simulink model "35 Bus Network Electricity Transmission Model"  (R2023b)
settings: Solver=VariableStepAuto  StartTime=0.0  StopTime=1  RelTol=1e-3
model workspace (MAT data in the model file):
  T_set = 0.0001
  Tp = 5e-05
undefined symbols (not defined in the file): D1, D11, Delta, DiscIntNeverNeededParam
libraries: spsSeriesRLCBranchLib x57, spsLoadFlowBusLib x35, spsThreePhaseSeriesRLCLoadLib x28, spsThreePhaseTransformerTwoWindingsLib x22, spsDistributedParametersLineLib x22, spsGenericPowerSystemStabilizerLib x20, spsThreePhaseVIMeasurementLib x14, spsSynchronousMachinepuStandardLib x10, spsExcitationSystemLib x10, spsHydraulicTurbineandGovernorLib x10, spsFourierLib x8, spsMeanLib x8
(part 3 of 8)

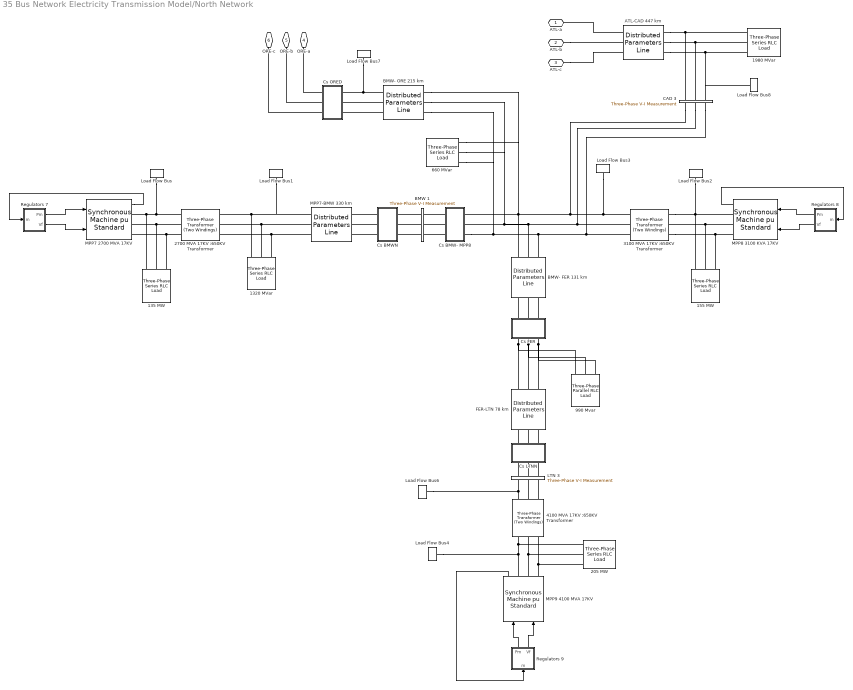
== system 35 Bus Network Electricity Transmission Model/North Network ==
  1320 MVar : spsThreePhaseSeriesRLCLoadLib/Three-Phase Series RLC Load  LConnTagsString=A|B|C  Configuration=Y (grounded)  NominalVoltage=650e3  Vabc=[1e3 1e3 1e3]  Vabcp=[1e3 1e3 1e3]  NominalFrequency=60  UnbalancedPower=off  ActivePower=4400e3  InductivePower=1320e6  CapacitivePower=0  Pabc=[10e3 9e3 11e3]  QLabc=[100 90 110]  QCabc=[100 90 110]  Pabcp=[10e3 9e3 11e3]  QLabcp=[100 90 110]  QCabcp=[100 90 110]  Measurements=None  LoadType=constant Z
  135 MW : spsThreePhaseSeriesRLCLoadLib/Three-Phase Series RLC Load  LConnTagsString=A|B|C  Configuration=Y (grounded)  NominalVoltage=17e3  Vabc=[1e3 1e3 1e3]  Vabcp=[1e3 1e3 1e3]  NominalFrequency=60  UnbalancedPower=off  ActivePower=135e6  InductivePower=0  CapacitivePower=0  Pabc=[10e3 9e3 11e3]  QLabc=[100 90 110]  QCabc=[100 90 110]  Pabcp=[10e3 9e3 11e3]  QLabcp=[100 90 110]  QCabcp=[100 90 110]  Measurements=None  LoadType=constant Z
  155 MW : spsThreePhaseSeriesRLCLoadLib/Three-Phase Series RLC Load  LConnTagsString=A|B|C  Configuration=Y (grounded)  NominalVoltage=17e3  Vabc=[1e3 1e3 1e3]  Vabcp=[1e3 1e3 1e3]  NominalFrequency=60  UnbalancedPower=off  ActivePower=155e6  InductivePower=0  CapacitivePower=0  Pabc=[10e3 9e3 11e3]  QLabc=[100 90 110]  QCabc=[100 90 110]  Pabcp=[10e3 9e3 11e3]  QLabcp=[100 90 110]  QCabcp=[100 90 110]  Measurements=None  LoadType=constant Z
  1980 MVar : spsThreePhaseSeriesRLCLoadLib/Three-Phase Series RLC Load  LConnTagsString=A|B|C  Configuration=Y (grounded)  NominalVoltage=650e3  Vabc=[1e3 1e3 1e3]  Vabcp=[1e3 1e3 1e3]  NominalFrequency=60  UnbalancedPower=off  ActivePower=6600e3  InductivePower=1980e6  CapacitivePower=0  Pabc=[10e3 9e3 11e3]  QLabc=[100 90 110]  QCabc=[100 90 110]  Pabcp=[10e3 9e3 11e3]  QLabcp=[100 90 110]  QCabcp=[100 90 110]  Measurements=None  LoadType=constant Z
  205 MW : spsThreePhaseSeriesRLCLoadLib/Three-Phase Series RLC Load  LConnTagsString=A|B|C  Configuration=Y (grounded)  NominalVoltage=17e3  Vabc=[1e3 1e3 1e3]  Vabcp=[1e3 1e3 1e3]  NominalFrequency=60  UnbalancedPower=off  ActivePower=205e6  InductivePower=0  CapacitivePower=0  Pabc=[10e3 9e3 11e3]  QLabc=[100 90 110]  QCabc=[100 90 110]  Pabcp=[10e3 9e3 11e3]  QLabcp=[100 90 110]  QCabcp=[100 90 110]  Measurements=None  LoadType=constant Z
  "2700 MVA 17KV :650KV Transformer " : spsThreePhaseTransformerTwoWindingsLib/Three-Phase Transformer (Two Windings)  Winding1Connection=Yg  Winding2Connection=Delta (D1)  CoreType=Three single-phase transformers  SetSaturation=off  Hysteresis=off  DataFile='hysteresis'  SetInitialFlux=off  Measurements=None  UNITS=pu  NominalPower=[ 2700e6 , 60 ]  Winding1=[650e3 , 0.002 , 0.08 ]  Winding2=[17e3 , 0.002 , 0.08 ]  Rm=500  Lm=500  L0=0.5  Saturation=[ 0,0 ; 0.0024,1.2 ; 1.0,1.52 ]  InitialFluxes=[ 0.8 , -0.8 , 0.7 ]  BreakLoop=off  DiscreteSolver=Trapezoidal iterative  DataType=off  TransfoNumber=1
  "3100 MVA 17KV :650KV Transformer " : spsThreePhaseTransformerTwoWindingsLib/Three-Phase Transformer (Two Windings)  Winding1Connection=Yg  Winding2Connection=Delta (D1)  CoreType=Three single-phase transformers  SetSaturation=off  Hysteresis=off  DataFile='hysteresis'  SetInitialFlux=off  Measurements=None  UNITS=pu  NominalPower=[ 3100e6 , 60 ]  Winding1=[ 650e3 , 0.002 , 0.08 ]  Winding2=[ 17e3 , 0.002 , 0.08 ]  Rm=500  Lm=500  L0=0.5  Saturation=[ 0,0 ; 0.0024,1.2 ; 1.0,1.52 ]  InitialFluxes=[ 0.8 , -0.8 , 0.7 ]  BreakLoop=off  DiscreteSolver=Trapezoidal iterative  DataType=off  TransfoNumber=1
  "4100 MVA 17KV :650KV Transformer " : spsThreePhaseTransformerTwoWindingsLib/Three-Phase Transformer (Two Windings)  Winding1Connection=Yg  Winding2Connection=Delta (D1)  CoreType=Three single-phase transformers  SetSaturation=off  Hysteresis=off  DataFile='hysteresis'  SetInitialFlux=off  Measurements=None  UNITS=pu  NominalPower=[ 4100e6 , 60 ]  Winding1=[ 650e3 , 0.002 , 0.08 ]  Winding2=[ 17e3 , 0.002 , 0.08 ]  Rm=500  Lm=500  L0=0.5  Saturation=[ 0,0 ; 0.0024,1.2 ; 1.0,1.52 ]  InitialFluxes=[ 0.8 , -0.8 , 0.7 ]  BreakLoop=off  DiscreteSolver=Trapezoidal iterative  DataType=off  TransfoNumber=1
  660 MVar : spsThreePhaseSeriesRLCLoadLib/Three-Phase Series RLC Load  LConnTagsString=A|B|C  Configuration=Y (grounded)  NominalVoltage=650e3  Vabc=[1e3 1e3 1e3]  Vabcp=[1e3 1e3 1e3]  NominalFrequency=60  UnbalancedPower=off  ActivePower=2200e3  InductivePower=660e6  CapacitivePower=0  Pabc=[10e3 9e3 11e3]  QLabc=[100 90 110]  QCabc=[100 90 110]  Pabcp=[10e3 9e3 11e3]  QLabcp=[100 90 110]  QCabcp=[100 90 110]  Measurements=None  LoadType=constant Z
  990 Mvar : spsThreePhaseParallelRLCLoadLib/Three-Phase Parallel RLC Load  LConnTagsString=A|B|C  Configuration=Y (grounded)  NominalVoltage=650e3  Vabc=[1e3 1e3 1e3]  Vabcp=[1e3 1e3 1e3]  NominalFrequency=60  UnbalancedPower=off  ActivePower=3300e3  InductivePower=990e6  CapacitivePower=0  Pabc=[10e3 9e3 11e3]  QLabc=[100 90 110]  QCabc=[100 90 110]  Pabcp=[10e3 9e3 11e3]  QLabcp=[100 90 110]  QCabcp=[100 90 110]  Measurements=None  LoadType=constant Z
  ATL-CAD 447 km : spsDistributedParametersLineLib/Distributed Parameters Line  Phases=3  Length=447  Frequency=60  Resistance=[0.01273 0.3864]/6  Inductance="[0.9337e-3  4.1264e-3]/6"  Capacitance=[12.74e-9 7.751e-9]*6  x1=[-0.00258 -5.31602971925857e-09 -148199.916502334 -96849.1917886608;-0.00252 -6.01655285993135e-09 -145971.498172148 -100176.353662668;-0.00246 -6.71399782098787e-09 -143668.398126254 -103452.263463096;-0.0024 -7.40800777669876e-09 -141291.794673192 -106675.245173957;-0.00234 -8.09822765874685e-09 -138842.903727203 -109843.649858256;-0.00228 -8.78430433788667e-09 -136322.978186145 -112955.85650161;-0.00222 -9.46588680461196e-09 -133733.307290488 -116010.272841594;-0.00216 -1.01426263487385e-08 -131075.215963714 -119005.336182368;-0.0021 -1.08141767378109e-08 -128350.064134461 -121939.514194186;-0.00204 -1.14801943942412e-08 -125559.246040761 -124811.305697358;-0.00198 -1.21403385710898e-08 -122704.189516718 -127619.241430289;-0.00192 -1.27942715263977e-08 -119786.355262006 -130361.884801171;-0.00186 -1.34416586959818e-08 -116807.236094544 -133037.832622978;-0.0018 -1.40821688646038e-08 -113768.356186747 -135645.715831359;-0.00174 -1.4715474335426e-08 -110671.270285727 -138184.200185075;-0.00168 -1.53412510976676e-08 -107517.562917858 -140651.986948627;-0.00162 -1.59591789923738e-08 -104308.847578105 -143047.813556706;-0.00156 -1.65689418762158e-08 -101046.765904525 -145370.454260149;-0.0015 -1.71702277832351e-08 -97732.9868383792 -147618.720753056;-0.00144 -1.77627290844512e-08 -94369.2057702685 -149791.462780745;-0.00138 -1.83461426452502e-08 -90957.1436727434 -151887.568728248;-0.00132 -1.89201699804741e-08 -87498.5462198204 -153905.96618903;-0.00126 -1.94845174071315e-08 -83995.1828938642 -155845.622513654;-0.0012 -2.00388961946509e-08 -80448.8460802869 -157705.545338104;-0.00114 -2.05830227126009e-08 -76861.3501505312 -159484.783091496;-0.00108 -2.11166185758005e-08 -73234.530533804 -161182.425482918;-0.00102 -2.16394107867466e-08 -69570.2427780372 -162797.603967154;-0.00096 -2.21511318752838e-08 -65870.3616005549 -164329.492189047;-0.0009 -2.26515200354478e-08 -62136.7799289334 -165777.306406276;-0.00084 -2.31403192594097e-08 -58371.4079325445 -167140.305890335;-0.00078 -2.36172794684545e-08 -54576.1720452778 -168417.793305503;-0.00072 -2.40821566409261e-08 -50753.013979941 -169609.115065613;-0.00066 -2.45347129370731e-08 -46903.8897348442 -170713.661668439;-0.0006 -2.49747168207321e-08 -43030.7685930748 -171730.86800753;-0.00054 -2.5401943177786e-08 -39135.632114976 -172660.213661326;-0.00048 -2.58161734313361e-08 -35220.4731243439 -173501.22315942;-0.00042 -2.62171956535308e-08 -31287.2946888618 -174253.466225811;-0.00036 -2.6604804673991e-08 -27338.1090952941 -174916.557999047;-0.0003 -2.69788021847797e-08 -23374.9368199632 -175490.159229125;-0.00024 -2.73389968418598e-08 -19399.8054950359 -175973.976451055;-0.00018 -2.7685204362989e-08 -15414.7488711503 -176367.762135008;-0.00012 -2.80172476220023e-08 -11421.8057769103 -176671.314812951;-6e-05 -2.8334956739433e-08 -7423.01907578413 -176884.479181725]  x2=[-0.00258 -4.87845949451141e-08 -272951.515548649 -95064.3825346825;-0.00252 -4.87524641140646e-08 -270731.542277713 -101213.579527017;-0.00246 -4.86953906215323e-08 -268373.057747203 -107310.993781853;-0.0024 -4.86134036673707e-08 -265877.268601386 -113353.505749391;-0.00234 -4.85065451976205e-08 -263245.451732106 -119338.023968856;-0.00228 -4.83748698830492e-08 -260478.953625503 -125261.486650145;-0.00222 -4.8218445091181e-08 -257579.189673127 -131120.863240298;-0.00216 -4.80373508518297e-08 -254547.643447798 -136913.155973982;-0.0021 -4.78316798161544e-08 -251385.865944582 -142635.401407206;-0.00204 -4.76015372092573e-08 -248095.474787272 -148284.67193347;-0.00198 -4.73470407763487e-08 -244678.153400783 -153858.077281588;-0.00192 -4.70683207225062e-08 -241135.650149882 -159352.765994398;-0.00186 -4.67655196460595e-08 -237469.77744469 -164765.926887624;-0.0018 -4.64387924656344e-08 -233682.41081342 -170094.790488131;-0.00174 -4.60883063408937e-08 -229775.487942824 -175336.630450834;-0.00168 -4.5714240587015e-08 -225751.007686833 -180488.764953549;-0.00162 -4.53167865829499e-08 -221611.02904391 -185548.558069065;-0.00156 -4.48961476735111e-08 -217357.670103628 -190513.421113731;-0.0015 -4.44525390653371e-08 -212993.106963013 -195380.813971871;-0.00144 -4.39861877167887e-08 -208519.572613215 -200148.24639536;-0.00138 -4.34973322218332e-08 -203939.35579707 -204813.27927768;-0.00132 -4.29862226879746e-08 -199254.799838133 -209373.525901806;-0.00126 -4.24531206082949e-08 -194468.301441793 -213826.653161304;-0.0012 -4.18982987276684e-08 -189582.309469075 -218170.382753982;-0.00114 -4.13220409032214e-08 -184599.323683754 -222402.492347517;-0.00108 -4.07246419591047e-08 -179521.893473433 -226520.816716443;-0.00102 -4.01064075356569e-08 -174352.616545228 -230523.248849912;-0.00096 -3.94676539330326e-08 -169094.137596732 -234407.74102969;-0.0009 -3.88087079493778e-08 -163749.146962942 -238172.305877801;-0.00084 -3.81299067136336e-08 -158320.379239828 -241815.017373306;-0.00078 -3.74315975130551e-08 -152810.611885272 -245334.011837695;-0.00072 -3.67141376155325e-08 -147222.66379806 -248727.488888376;-0.00066 -3.59778940868065e-08 -141559.393875686 -251993.712359787;-0.0006 -3.52232436026707e-08 -135823.699551689 -255131.011191646;-0.00054 -3.4450572256257e-08 -130018.515313268 -258137.7802839;-0.00048 -3.36602753605036e-08 -124146.811199946 -261012.481317923;-0.00042 -3.28527572459055e-08 -118211.591284045 -263753.643543548;-0.00036 -3.20284310536511e-08 -112215.892133745 -266359.864531529;-0.0003 -3.11877185242524e-08 -106162.781259517 -268829.810891052;-0.00024 -3.03310497817739e-08 -100055.355544735 -271162.218951918;-0.00018 -2.94588631137736e-08 -93896.739661245 -273355.895411067;-0.00012 -2.85716047470672e-08 -87690.0844707324 -275409.717943088;-6e-05 -2.76697286194296e-08 -81438.5654126781 -277322.635774423]  x3=[-0.00258 -2.63643710027556e-10 -3962.84356104863 3839.79887558329;-0.00252 -2.75977166927134e-10 -4048.67593368483 3749.18694624542;-0.00246 -2.8816942880864e-10 -4132.43692890242 3656.65686358885;-0.0024 -3.00214257885608e-10 -4214.08369302854 3562.25596771361;-0.00234 -3.12105491800921e-10 -4293.57445406998 3466.03255586237;-0.00228 -3.23837046779582e-10 -4370.86854308459 3368.03585771063;-0.00222 -3.3540292074129e-10 -4445.92641498819 3268.31601017994;-0.00216 -3.46797196371213e-10 -4518.70966878661 3166.92403178691;-0.0021 -3.58014044147398e-10 -4589.18106722233 3063.91179654118;-0.00204 -3.69047725323257e-10 -4657.30455582573 2959.33200740577;-0.00198 -3.79892594863624e-10 -4723.04528136129 2853.23816933319;-0.00192 -3.9054310433285e-10 -4786.36960965905 2745.68456189141;-0.00186 -4.00993804733492e-10 -4847.24514282257 2636.72621149335;-0.0018 -4.11239349294119e-10 -4905.64073580424 2526.41886324438;-0.00174 -4.21274496204818e-10 -4961.52651233964 2414.81895242213;-0.00168 -4.31094111299001e-10 -5014.87388023287 2301.9835756031;-0.00162 -4.4069317068014e-10 -5065.65554598475 2187.97046145102;-0.00156 -4.50066763292085e-10 -5113.84552875675 2072.83794118182;-0.0015 -4.59210093431653e-10 -5159.41917366325 1956.64491872026;-0.00144 -4.68118483202194e-10 -5202.35316438539 1839.45084056365;-0.00138 -4.76787374906894e-10 -5242.62553510019 1721.31566536786;-0.00132 -4.85212333380574e-10 -5280.21568171866 1602.29983327142;-0.00126 -4.93389048258803e-10 -5315.10437242719 1482.46423497317;-0.0012 -5.01313336183161e-10 -5347.27375752696 1361.87018057953;-0.00114 -5.08981142941523e-10 -5376.70737856611 1240.57936823703;-0.00108 -5.16388545542266e-10 -5403.39017676026 1118.65385256647;-0.00102 -5.23531754221346e-10 -5427.30850069681 996.156012914591;-0.00096 -5.30407114381212e-10 -5448.45011331927 873.148521439658;-0.0009 -5.37011108460564e-10 -5466.80419818797 749.694311047227;-0.00084 -5.43340357734003e-10 -5482.36136501396 625.856543192506;-0.00078 -5.4939162404065e-10 -5495.11365446321 501.698575565788;-0.00072 -5.55161811440848e-10 -5505.05454222881 377.283929677488;-0.00066 -5.60647967800102e-10 -5512.1789423689 252.676258359358;-0.0006 -5.65847286299446e-10 -5516.48320990871 127.939313198532;-0.00054 -5.70757106871463e-10 -5517.96514270545 3.13691192102679;-0.00048 -5.75374917561226e-10 -5516.6239825749 -121.667094258581;-0.00042 -5.79698355811459e-10 -5512.46041567938 -246.408853304616;-0.00036 -5.83725209671265e-10 -5505.47657217664 -371.024545028189;-0.0003 -5.87453418927801e-10 -5495.67602513006 -495.45041373878;-0.00024 -5.90881076160322e-10 -5483.06378868061 -619.622800862831;-0.00018 -5.94006427716053e-10 -5467.6463154815 -743.478177512648;-0.00012 -5.96827874607388e-10 -5449.43149339691 -866.953176988952;-6e-05 -5.99343973329962e-10 -5428.42864146637 -989.984627200456]  x4=[-0.00258 1.25550589079962e-11 -6479.77720814425 -5262.43401290687;-0.00252 1.56860264672874e-11 -6359.09575517457 -5407.6451916609;-0.00246 1.88089687655935e-11 -6235.16087131396 -5550.08971921309;-0.0024 2.19222880479294e-11 -6108.03596393906 -5689.69471831107;-0.00234 2.50243914826226e-11 -5977.78607250148 -5826.38876445768;-0.00228 2.81136919762357e-11 -5844.47783525243 -5960.10192245311;-0.00222 3.11886089855525e-11 -5708.17945514932 -6090.765782175;-0.00216 3.42475693262131e-11 -5568.96066496193 -6218.31349357831;-0.0021 3.7289007977584e-11 -5426.89269159579 -6342.67980089709;-0.00204 4.0311368883452e-11 -5282.04821965117 -6463.80107603048;-0.00198 4.33131057481307e-11 -5134.50135423636 -6581.61535109605;-0.00192 4.62926828275745e-11 -4984.32758305404 -6696.06235013374;-0.00186 4.92485757150933e-11 -4831.60373778045 -6807.0835199441;-0.0018 5.21792721212672e-11 -4676.40795475683 -6914.62206004521;-0.00174 5.50832726476618e-11 -4518.81963501348 -7018.62295173288;-0.00168 5.7959091553948e-11 -4358.91940364667 -7119.0329862292;-0.00162 6.08052575180343e-11 -4196.78906856938 -7215.80079190516;-0.00156 6.36203143888224e-11 -4032.51157865687 -7308.87686056331;-0.0015 6.64028219312009e-11 -3866.17098130847 -7398.21357276708;-0.00144 6.91513565628964e-11 -3697.85237944741 -7483.76522220376;-0.00138 7.18645120828041e-11 -3527.64188798056 -7565.48803906867;-0.00132 7.45409003904268e-11 -3355.6265897405 -7643.34021245865;-0.00126 7.71791521960522e-11 -3181.89449093227 -7717.28191176325;-0.0012 7.97779177213074e-11 -3006.53447610784 -7787.27530704281;-0.00114 8.23358673897299e-11 -2829.63626269106 -7853.28458838299;-0.00108 8.4851692507004e-11 -2651.29035507662 -7915.27598421574;-0.00102 8.73241059305124e-11 -2471.58799832631 -7973.21777859748;-0.00096 8.97518427278629e-11 -2290.62113148636 -8027.08032743556;-0.0009 9.21336608240504e-11 -2108.48234054972 -8076.83607365474;-0.00084 9.4468341636926e-11 -1925.26481108739 -8122.45956129586;-0.00078 9.67546907006459e-11 -1741.06228057291 -8163.92744853963;-0.00072 9.89915382767822e-11 -1555.96899042455 -8201.21851964869;-0.00066 1.01177739952783e-10 -1370.07963778969 -8234.31369582201;-0.0006 1.03312177227474e-10 -1183.48932709597 -8263.19604495592;-0.00054 1.05393758083306e-10 -996.293521394147 -8287.85079030692;-0.00048 1.0742141754505e-10 -808.587993517389 -8308.26531805173;-0.00042 1.09394118224658e-10 -620.468777082158 -8324.42918374073;-0.00036 1.11310850852011e-10 -432.032117355627 -8336.33411764156;-0.0003 1.13170634791281e-10 -243.374422014822 -8343.97402897006;-0.00024 1.14972518542639e-10 -54.5922118226712 -8347.34500900643;-0.00018 1.16715580229062e-10 134.217928753796 -8346.44533309499;-0.00012 1.18398928067984e-10 322.95940095785 -8341.27546152656;-6e-05 1.20021700827546e-10 511.535641164771 -8331.83803930296]  x5=0.00252797080447097  V1=[6.404e-19 2.341e-08 2.341e-08;377 377 377;-1.588 0.8733 -0.6975]  V2=[3.447e-16 8.016e-05 8.016e-05;377 377 377;2.581 0.8892 -0.6816]  I1=[4.995e-19 5.332e-07 5.332e-07;377 377 377;1.203 -0.6479 -2.219]  I2=[4.022e-19 5.225e-07 5.225e-07;377 377 377;-2.95 1.909 0.3385]  nHarmo=1  Measurements=None  Decoupling=off  VsMag0=0  VrMag0=0  VsAngle0=0  VrAngle0=0  IsMag0=0  IrMag0=0  IsAngle0=0  IrAngle0=0
      settings: LibrarySourceBlock=sps_lib/Power Grid Elements/Distributed Parameters Line
  BMW 1 : spsThreePhaseVIMeasurementLib/Three-Phase V-I Measurement  VoltageMeasurement=no  SetLabelV=off  LabelV=Vabc  Vpu=off  VpuLL=off  CurrentMeasurement=no  SetLabelI=off  LabelI=Iabc  Ipu=off  Pbase=100e6  Vbase=500e3  OutputType=Complex  PhasorSimulation=off  PSBequivalent=0
  BMW- FER 131 km : spsDistributedParametersLineLib/Distributed Parameters Line  Phases=3  Length=131  Frequency=60  Resistance=[0.01273 0.3864]/6  Inductance="[0.9337e-3  4.1264e-3]/6"  Capacitance=[12.74e-9 7.751e-9]*6  x1=[-0.00078 -2.36172794684545e-08 -54576.1720452778 -168417.793305503;-0.00072 -2.40821566409261e-08 -50753.013979941 -169609.115065613;-0.00066 -2.45347129370731e-08 -46903.8897348442 -170713.661668439;-0.0006 -2.49747168207321e-08 -43030.7685930748 -171730.86800753;-0.00054 -2.5401943177786e-08 -39135.632114976 -172660.213661326;-0.00048 -2.58161734313361e-08 -35220.4731243439 -173501.22315942;-0.00042 -2.62171956535308e-08 -31287.2946888618 -174253.466225811;-0.00036 -2.6604804673991e-08 -27338.1090952941 -174916.557999047;-0.0003 -2.69788021847797e-08 -23374.9368199632 -175490.159229125;-0.00024 -2.73389968418598e-08 -19399.8054950359 -175973.976451055;-0.00018 -2.7685204362989e-08 -15414.7488711503 -176367.762135008;-0.00012 -2.80172476220023e-08 -11421.8057769103 -176671.314812951;-6e-05 -2.8334956739433e-08 -7423.01907578413 -176884.479181725]  x2=[-0.00078 -3.00128995055536e-08 -18133.3222512837 -146952.987792149;-0.00072 -3.02085545374644e-08 -14804.9695526073 -147325.549479172;-0.00066 -3.03887543146839e-08 -11469.0423579434 -147622.736692817;-0.0006 -3.05534066436764e-08 -8127.24738928558 -147844.397386617;-0.00054 -3.0702427285268e-08 -4781.29437068918 -147990.418154863;-0.00048 -3.08357399977448e-08 -1432.89515354457 -148060.724290632;-0.00042 -3.09532765758598e-08 1916.23715923744 -148055.279824007;-0.00036 -3.10549768857278e-08 5264.38908968081 -147974.087540477;-0.0003 -3.1140788895591e-08 8609.84766139116 -147817.188979514;-0.00024 -3.12106687024397e-08 11950.9012759463 -147584.664413322;-0.00018 -3.12645805544733e-08 15285.8405885813 -147276.632805765;-0.00012 -3.13024968693923e-08 18612.9593827214 -146893.251751505;-6e-05 -3.13243982485092e-08 21930.5554429133 -146434.717395374]  x3=[-0.00078 -5.25941512392795e-10 1443.1371085866 -8256.16688772562;-0.00072 -5.32217136019589e-10 1629.50173084287 -8221.41547476303;-0.00066 -5.38220467525353e-10 1815.03266990392 -8182.45783372926;-0.0006 -5.43948435494761e-10 1999.6350047131 -8139.31389607332;-0.00054 -5.49398109393558e-10 2183.21428930486 -8092.00573503091;-0.00048 -5.5456670106788e-10 2365.67660112505 -8040.55755433139;-0.00042 -5.59451566170721e-10 2546.92858908342 -7984.99567581466;-0.00036 -5.64050205514833e-10 2726.87752131379 -7925.34852596442;-0.0003 -5.68360266351354e-10 2905.43133261735 -7861.64662136469;-0.00024 -5.72379543573519e-10 3082.49867156495 -7793.92255308695;-0.00018 -5.76105980844834e-10 3257.98894723415 -7722.21097001592;-0.00012 -5.79537671651134e-10 3431.81237555723 -7646.54856112257;-6e-05 -5.82672860275993e-10 3603.88002525638 -7566.97403669339]  x4=[-0.00078 1.38256010660376e-10 -3642.04661389476 1435.98650461832;-0.00072 1.38062119582989e-10 -3673.59294614646 1353.24476886254;-0.00066 1.37797593374128e-10 -3703.25980036671 1269.81068807791;-0.0006 1.3746256737029e-10 -3731.03199844472 1185.72694868187;-0.00054 1.37057212976969e-10 -3756.89533161078 1101.03656946917;-0.00048 1.36581737580963e-10 -3780.83656770575 1015.7828796027;-0.00042 1.3603638444427e-10 -3802.84345795085 930.009496445527;-0.00036 1.35421432579632e-10 -3822.90474321439 843.76030324537;-0.0003 1.34737196607786e-10 -3841.01015977215 757.079426683174;-0.00024 1.33984026596498e-10 -3857.15044455846 670.011214297068;-0.00018 1.33162307881464e-10 -3871.31733990539 582.600211793343;-0.00012 1.32272460869161e-10 -3883.5035977675 494.891140256051;-6e-05 1.31314940821763e-10 -3893.70298343011 406.928873266868]  x5=0.000740859452764423  V1=[1.271e-18 2.341e-08 2.341e-08;377 377 377;2.226 1.284 -0.2866]  V2=[3.351e-20 3.07e-09 3.07e-09;377 377 377;-0.6702 -1.817 2.896]  I1=[5.66e-21 5.705e-10 5.705e-10;377 377 377;-2.518 2.745 1.174]  I2=[6.071e-21 5.74e-10 5.74e-10;377 377 377;0.8934 -0.2657 -1.836]  nHarmo=1  Measurements=None  Decoupling=off  VsMag0=0  VrMag0=0  VsAngle0=0  VrAngle0=0  IsMag0=0  IrMag0=0  IsAngle0=0  IrAngle0=0
      settings: LibrarySourceBlock=sps_lib/Power Grid Elements/Distributed Parameters Line
  BMW- ORE 215 km : spsDistributedParametersLineLib/Distributed Parameters Line  Phases=3  Length=215  Frequency=60  Resistance=[0.01273 0.3864]/6  Inductance="[0.9337e-3  4.1264e-3]/6"  Capacitance=[12.74e-9 7.751e-9]*6  x1=[-0.00126 -1.94845174071315e-08 -83995.1828938642 -155845.622513654;-0.0012 -2.00388961946509e-08 -80448.8460802869 -157705.545338104;-0.00114 -2.05830227126009e-08 -76861.3501505312 -159484.783091496;-0.00108 -2.11166185758005e-08 -73234.530533804 -161182.425482918;-0.00102 -2.16394107867466e-08 -69570.2427780372 -162797.603967154;-0.00096 -2.21511318752838e-08 -65870.3616005549 -164329.492189047;-0.0009 -2.26515200354478e-08 -62136.7799289334 -165777.306406276;-0.00084 -2.31403192594097e-08 -58371.4079325445 -167140.305890335;-0.00078 -2.36172794684545e-08 -54576.1720452778 -168417.793305503;-0.00072 -2.40821566409261e-08 -50753.013979941 -169609.115065613;-0.00066 -2.45347129370731e-08 -46903.8897348442 -170713.661668439;-0.0006 -2.49747168207321e-08 -43030.7685930748 -171730.86800753;-0.00054 -2.5401943177786e-08 -39135.632114976 -172660.213661326;-0.00048 -2.58161734313361e-08 -35220.4731243439 -173501.22315942;-0.00042 -2.62171956535308e-08 -31287.2946888618 -174253.466225811;-0.00036 -2.6604804673991e-08 -27338.1090952941 -174916.557999047;-0.0003 -2.69788021847797e-08 -23374.9368199632 -175490.159229125;-0.00024 -2.73389968418598e-08 -19399.8054950359 -175973.976451055;-0.00018 -2.7685204362989e-08 -15414.7488711503 -176367.762135008;-0.00012 -2.80172476220023e-08 -11421.8057769103 -176671.314812951;-6e-05 -2.8334956739433e-08 -7423.01907578413 -176884.479181725]  x2=[-0.00126 1.9689198857407e-09 -171164.695620357 -165669.545679999;-0.0012 1.63120802744188e-09 -167373.861811592 -169498.519608373;-0.00114 1.29266161297497e-09 -163497.39644241 -173240.774962143;-0.00108 9.53453848941217e-10 -159537.282784125 -176894.397134321;-0.00102 6.13758280300546e-10 -155495.546904056 -180457.516864292;-0.00096 2.73748701582723e-10 -151374.256628965 -183928.311194165;-0.0009 -6.64009320291239e-11 -147175.520487107 -187305.004401425;-0.00084 -4.06516593697196e-10 -142901.486629477 -190585.868907436;-0.00078 -7.4642427396437e-10 -138554.341730772 -193769.226161291;-0.00072 -1.08595006978065e-09 -134136.309870647 -196853.447498599;-0.00066 -1.42492027347518e-09 -129649.651395838 -199836.954974732;-0.0006 -1.7631614616283e-09 -125096.661763725 -202718.222172139;-0.00054 -2.10050058379817e-09 -120479.670367934 -205495.77498128;-0.00048 -2.43676505105659e-09 -115801.039346574 -208168.192354815;-0.00042 -2.77178282428864e-09 -111063.162373726 -210734.107034636;-0.00036 -3.10538250221113e-09 -106268.463434798 -213192.206251379;-0.0003 -3.43739340906461e-09 -101419.39558636 -215541.232396065;-0.00024 -3.76764568193429e-09 -96518.4397011257 -217779.983663513;-0.00018 -4.09597035765501e-09 -91568.1031986844 -219907.314667207;-0.00012 -4.42219945925592e-09 -86570.9187626627 -221922.137025298;-6e-05 -4.74616608190062e-09 -81529.4430449554 -223823.419917437]  x3=[-0.00126 -1.80150237413883e-10 -3362.58932738102 3762.49944929283;-0.0012 -1.76212447887123e-10 -3446.82705388805 3685.48334361674;-0.00114 -1.72184504815992e-10 -3529.30131998427 3606.58167656216;-0.00108 -1.68068468970593e-10 -3609.96993031119 3525.83481567987;-0.00102 -1.63866446190921e-10 -3688.79161331719 3443.28407255596;-0.00096 -1.59580586309473e-10 -3765.72604237279 3358.97168167594;-0.0009 -1.5521308205136e-10 -3840.73385640249 3272.94077881692;-0.00084 -1.50766167912461e-10 -3913.77668002265 3185.23537897847;-0.00078 -1.46242119016219e-10 -3984.81714317504 3095.90035386375;-0.00072 -1.41643249949645e-10 -4053.81890024602 3004.98140892233;-0.00066 -1.36971913579131e-10 -4120.74664866168 2912.52505996643;-0.0006 -1.32230499846679e-10 -4185.56614694924 2818.57860937258;-0.00054 -1.27421434547168e-10 -4248.24423225564 2723.19012188083;-0.00048 -1.22547178087264e-10 -4308.7488373143 2626.40840000396;-0.00042 -1.1761022422664e-10 -4367.04900685127 2528.2829590592;-0.00036 -1.12613098802114e-10 -4423.11491342254 2428.86400183528;-0.0003 -1.0755835843539e-10 -4476.91787267433 2328.20239290778;-0.00024 -1.02448589225041e-10 -4528.43035801854 2226.34963261584;-0.00018 -9.72864054234115e-11 -4577.62601471581 2123.35783071364;-0.00012 -9.20744480991217e-11 -4624.47967335915 2019.2796797101;-6e-05 -8.68153837858442e-11 -4668.96736275104 1914.16842791042]  x4=[-0.00126 1.21169041062424e-10 -3247.07632241657 -10042.5119136274;-0.0012 1.09690864843295e-10 -3019.10882125781 -10113.3848460686;-0.00114 9.8156568750857e-11 -2789.59668823938 -10179.0835839487;-0.00108 8.65720539441217e-11 -2558.65734600942 -10239.5745145794;-0.00102 7.4943247274921e-11 -2326.4089474027 -10294.8266896829;-0.00096 6.32760982556224e-11 -2092.97031499138 -10344.8118412254;-0.0009 5.15765760152484e-11 -1858.46088029327 -10389.5043958798;-0.00084 3.98506662455594e-11 -1623.0006226684 -10428.8814881093;-0.00078 2.81043681386636e-11 -1386.71000793537 -10462.922971866;-0.00072 1.6343691317719e-11 -1149.70992673882 -10491.6114308976;-0.00066 4.57465276229953e-12 -912.12163269955 -10514.9321876585;-0.0006 -7.19672627000299e-12 -674.066680378925 -10532.8733108185;-0.00054 -1.89644233241655e-11 -435.666863089298 -10545.4256213677;-0.00048 -3.07224178289332e-11 -197.044150582316 -10552.5826973118;-0.00042 -4.24646941770546e-11 41.6793733530605 -10554.3408769588;-0.00036 -5.41852448029776e-11 280.381573350883 -10550.6992607913;-0.0003 -6.58780732564312e-11 518.940324954924 -10541.6597119274;-0.00024 -7.75371972703201e-11 757.233577099804 -10527.2268551675;-0.00018 -8.91566518213627e-11 995.139414554571 -10507.4080746276;-0.00012 -1.00730492181908e-10 1232.53612029679 -10482.2135099622;-6e-05 -1.12252796961368e-10 1469.30223778522 -10451.6560511761]  x5=0.00121591436904085  V1=[1.271e-18 2.341e-08 2.341e-08;377 377 377;2.047 1.175 -0.3959]  V2=[2.813e-15 0.004697 0.004697;377 377 377;-0.9882 1.143 -0.4279]  I1=[7.991e-18 6.252e-05 6.252e-05;377 377 377;-2.327 -0.3924 -1.963]  I2=[7.132e-18 6.19e-05 6.19e-05;377 377 377;0.3426 2.469 0.8982]  nHarmo=1  Measurements=None  Decoupling=off  VsMag0=0  VrMag0=0  VsAngle0=0  VrAngle0=0  IsMag0=0  IrMag0=0  IsAngle0=0  IrAngle0=0
      settings: LibrarySourceBlock=sps_lib/Power Grid Elements/Distributed Parameters Line
  CAD 3 : spsThreePhaseVIMeasurementLib/Three-Phase V-I Measurement  VoltageMeasurement=no  SetLabelV=off  LabelV=Vabc  Vpu=off  VpuLL=off  CurrentMeasurement=no  SetLabelI=off  LabelI=Iabc  Ipu=off  Pbase=100e6  Vbase=500e3  OutputType=Complex  PhasorSimulation=off  PSBequivalent=0
  Cs BMW- MPP8 : Subsystem
  Cs BMWN : Subsystem
  Cs FER : Subsystem
  Cs LTNN : Subsystem
  Cs ORED : Subsystem
  FER-LTN 78 km : spsDistributedParametersLineLib/Distributed Parameters Line  Phases=3  Length=78  Frequency=60  Resistance=[0.01273 0.3864]/6  Inductance="[0.9337e-3  4.1264e-3]/6"  Capacitance=[12.74e-9 7.751e-9]*6  x1=[-0.00048 -3.05426738644595e-08 0 0;-0.00042 -3.07047444550503e-08 0 0;-0.00036 -3.08511059310195e-08 0 0;-0.0003 -3.09816834111315e-08 -12885.8748975685 -169381.852854286;-0.00024 -3.10964100895346e-08 -9051.58214360524 -169629.99500703;-0.00018 -3.11952272699403e-08 -5212.65843296332 -169791.351319927;-0.00012 -3.12780843956533e-08 -1371.06782994823 -169865.839240105;-6e-05 -3.13449390754368e-08 2471.22423670307 -169853.420658168]  x2=[-0.00048 -3.37391762227311e-08 0 0;-0.00042 -3.37430146195138e-08 0 0;-0.00036 -3.37295894665179e-08 0 0;-0.0003 -3.36989076322998e-08 6092.64393193445 -152516.417752119;-0.00024 -3.36509848142529e-08 9540.6264547602 -152339.624598957;-0.00018 -3.35858455305762e-08 12983.7278168012 -152084.891678938;-0.00012 -3.3503523107731e-08 16420.1864637794 -151752.34931813;-6e-05 -3.340405966339e-08 19848.2442399526 -151342.167651349]  x3=[-0.00048 -5.92893739767097e-10 0 0;-0.00042 -5.96030232263695e-10 0 0;-0.00036 -5.98861784680094e-10 0 0;-0.0003 -6.01386948341758e-10 3354.90337281565 -7738.00376158879;-0.00024 -6.03604431328297e-10 3529.05919134546 -7660.14534710868;-0.00018 -6.05513099134441e-10 3701.40947798346 -7578.36786072577;-0.00012 -6.07111975250471e-10 3871.86605513834 -7492.71314131317;-6e-05 -6.08400241661825e-10 4040.34171407556 -7403.22501140806]  x4=[-0.00048 8.78780192191126e-11 0 0;-0.00042 8.87620207749491e-11 0 0;-0.00036 8.96006100408235e-11 0 0;-0.0003 9.03933579789721e-11 -3866.4677861276 630.952755869019;-0.00024 9.11398590049015e-11 -3879.74888822993 543.3410054975;-0.00018 9.1839731194893e-11 -3891.04503911153 455.451271827782;-0.00012 9.2492616481402e-11 -3900.35045945287 367.328520871624;-6e-05 9.30981808362522e-11 -3907.66038842897 279.017837856737]  x5=0.000441122422256679  V1=[6.391e-24 5.815e-13 5.815e-13;377 377 377;2.579 1.39 -0.1804]  V2=[2.845e-25 1.398e-13 1.398e-13;377 377 377;-0.3188 -1.706 3.006]  I1=[5.031e-26 2.613e-14 2.613e-14;377 377 377;-2.041 2.924 1.353]  I2=[5.244e-26 2.622e-14 2.622e-14;377 377 377;1.254 -0.1553 -1.726]  nHarmo=1  Measurements=None  Decoupling=off  VsMag0=0  VrMag0=0  VsAngle0=0  VrAngle0=0  IsMag0=0  IrMag0=0  IsAngle0=0  IrAngle0=0
      settings: LibrarySourceBlock=sps_lib/Power Grid Elements/Distributed Parameters Line
  LTN 3 : spsThreePhaseVIMeasurementLib/Three-Phase V-I Measurement  VoltageMeasurement=no  SetLabelV=off  LabelV=Vabc  Vpu=off  VpuLL=off  CurrentMeasurement=no  SetLabelI=off  LabelI=Iabc  Ipu=off  Pbase=100e6  Vbase=500e3  OutputType=Complex  PhasorSimulation=off  PSBequivalent=0
  Load Flow Bus : spsLoadFlowBusLib/Load Flow Bus  LConnTagsString=a  Phases=single  Connectors=on one side  ID=BUS_13  Vbase=17e3  Vref=1  Vangle=0  VLF=1  VLFb=1  VLFc=1  angleLF=0  angleLFb=0  angleLFc=0
  Load Flow Bus1 : spsLoadFlowBusLib/Load Flow Bus  LConnTagsString=a  Phases=single  Connectors=on one side  ID=BUS_14  Vbase=650e3  Vref=1  Vangle=0  VLF=1  VLFb=1  VLFc=1  angleLF=0  angleLFb=0  angleLFc=0
  Load Flow Bus2 : spsLoadFlowBusLib/Load Flow Bus  LConnTagsString=a  Phases=single  Connectors=on one side  ID=BUS_15  Vbase=17e3  Vref=1  Vangle=0  VLF=1  VLFb=1  VLFc=1  angleLF=0  angleLFb=0  angleLFc=0
  Load Flow Bus3 : spsLoadFlowBusLib/Load Flow Bus  LConnTagsString=a  Phases=single  Connectors=on one side  ID=BUS_16  Vbase=650e3  Vref=1  Vangle=0  VLF=1  VLFb=1  VLFc=1  angleLF=0  angleLFb=0  angleLFc=0
  Load Flow Bus4 : spsLoadFlowBusLib/Load Flow Bus  LConnTagsString=a  Phases=single  Connectors=on one side  ID=BUS_17  Vbase=17e3  Vref=1  Vangle=0  VLF=1  VLFb=1  VLFc=1  angleLF=0  angleLFb=0  angleLFc=0
  Load Flow Bus6 : spsLoadFlowBusLib/Load Flow Bus  LConnTagsString=a  Phases=single  Connectors=on one side  ID=BUS_18  Vbase=650e3  Vref=1  Vangle=0  VLF=1  VLFb=1  VLFc=1  angleLF=0  angleLFb=0  angleLFc=0
  Load Flow Bus7 : spsLoadFlowBusLib/Load Flow Bus  LConnTagsString=a  Phases=single  Connectors=on one side  ID=BUS_19  Vbase=650e3  Vref=1  Vangle=0  VLF=1  VLFb=1  VLFc=1  angleLF=0  angleLFb=0  angleLFc=0
  Load Flow Bus8 : spsLoadFlowBusLib/Load Flow Bus  LConnTagsString=a  Phases=single  Connectors=on one side  ID=BUS_20  Vbase=650e3  Vref=1  Vangle=0  VLF=1  VLFb=1  VLFc=1  angleLF=0  angleLFb=0  angleLFc=0
  MPP7 2700 MVA 17KV : spsSynchronousMachinepuStandardLib/Synchronous Machine pu Standard  PresetModel=No  MechanicalLoad=Mechanical power Pm  ShowDetailedParameters=on  RotorType=Salient-pole  Units=per unit standard parameters  MeasurementBus=off  NominalParameters=[2700e6 17000 60]  Reactances1=[ 1.81, 0.3, 0.23, 1.76, 0.65, 0.25, 0.15 ]  Reactances2=[ 1.305, 0.296, 0.252, 0.474, 0.243, 0.18 ]  dAxisTimeConstants=Short-circuit  qAxisTimeConstants=Open-circuit  TimeConstants1="[ 4.4849  0.0681  0.1  ]"  TimeConstants2=[ 8.0, 0.03, 1.0, 0.07 ]  TimeConstants3="[  4.49  0.0681  0.0513  ]"  TimeConstants4=[ 8.0, 0.03, 0.3371, 0.0295 ]  TimeConstants5=[ 1.01, 0.053, 0.1 ]  TimeConstants6=[ 1.3201, 0.023, 1.0, 0.07 ]  TimeConstants7=[0.012 0.003 0.003]  TimeConstants8=[ 1.3201, 0.0231, 0.3371, 0.0295 ]  StatorResistance=2.8544e-3  Mechanical=[3.5 0 32]  PolePairs=20  InitialConditions=[0 -81.9543 0.907703 0.907703 0.907703 -8.76021 -128.76 111.24 1.25655]  SetSaturation=off  Saturation=[0.6404,0.7127,0.8441,0.9214,0.9956,1.082,1.19,1.316,1.457;0.7,0.7698,0.8872,0.9466,0.9969,1.046,1.1,1.151,1.201]  LoadFlowParameters=[1,0,0,0,0]  TsPowergui=0  TsBlock=-1  IterativeModel=Trapezoidal non iterative  IterativeDiscreteModel=Trapezoidal non iterative  BusType=PV  Pref=2200e6  Qref=0  Qmin=-inf  Qmax=inf  PLF=0  QLF=0
  MPP7-BMW 330 km : spsDistributedParametersLineLib/Distributed Parameters Line  Phases=3  Length=330  Frequency=60  Resistance=[0.01273 0.3864]/6  Inductance="[0.9337e-3  4.1264e-3]/6"  Capacitance=[12.74e-9 7.751e-9]*6  x1=[-0.00192 1.03724074911367e-07 0 0;-0.00186 1.02350092033477e-07 0 0;-0.0018 1.0092374495729e-07 0 0;-0.00174 9.94457634283261e-08 0 0;-0.00168 9.79169036092462e-08 0 0;-0.00162 9.63379476929835e-08 0 0;-0.00156 9.47097035025604e-08 0 0;-0.0015 9.30330040777913e-08 0 0;-0.00144 9.13087072490838e-08 0 0;-0.00138 8.95376951985567e-08 0 0;-0.00132 8.77208740086996e-08 0 0;-0.00126 8.58591731988043e-08 0 0;-0.0012 8.39535452494054e-08 0 0;-0.00114 8.20049651149737e-08 -106157.296693431 -166257.140292923;-0.00108 8.00144297251117e-08 -102369.807162936 -168615.653864206;-0.00102 7.79829574745057e-08 -98529.9433475204 -170887.900551314;-0.00096 7.59115877018963e-08 -94639.6697924641 -173072.717830854;-0.0009 7.38013801583337e-08 -90700.9768336019 -175168.987909935;-0.00084 7.16534144649895e-08 -86715.8795790304 -177175.638298051;-0.00078 6.94687895608021e-08 -82686.4168781409 -179091.642355785;-0.00072 6.72486231402397e-08 -78614.6502785073 -180916.019820056;-0.00066 6.49940510814671e-08 -74502.6629711595 -182647.837305644;-0.0006 6.27062268652092e-08 -70352.5587247847 -184286.208782722;-0.00054 6.03863209846093e-08 -66166.4608094005 -185830.296030169;-0.00048 5.80355203463827e-08 -61946.5109100506 -187279.309064418;-0.00042 5.56550276635738e-08 -57694.8680310792 -188632.506543626;-0.00036 5.32460608402255e-08 -53413.7073915445 -189889.196146958;-0.0003 5.08098523482773e-08 -49105.2193123364 -191048.734928792;-0.00024 4.83476485970096e-08 -44771.6080955681 -192110.529647663;-0.00018 4.58607092953578e-08 -40415.0908968138 -193074.037069771;-0.00012 4.33503068074221e-08 -36037.8965907718 -193938.764246916;-6e-05 4.08177255015021e-08 -31642.2646309301 -194704.268768696]  x2=[-0.00192 1.00958472491216e-07 0 0;-0.00186 1.00656393299685e-07 0 0;-0.0018 1.00302816437425e-07 0 0;-0.00174 9.98979228008924e-08 0 0;-0.00168 9.94419195411539e-08 0 0;-0.00162 9.89350399579027e-08 0 0;-0.00156 9.83775433800997e-08 0 0;-0.0015 9.77697150332954e-08 0 0;-0.00144 9.71118658937035e-08 0 0;-0.00138 9.64043325290994e-08 0 0;-0.00132 9.56474769266262e-08 0 0;-0.00126 9.48416863075951e-08 0 0;-0.0012 9.39873729293762e-08 0 0;-0.00114 9.30849738744797e-08 -44025.6488640691 -141402.182108513;-0.00108 9.21349508269364e-08 -40816.2148713668 -142361.784066803;-0.00102 9.11377898360919e-08 -37585.8985489394 -143248.551105822;-0.00096 9.00940010679346e-08 -34336.3525863068 -144062.029539165;-0.0009 8.90041185440851e-08 -31069.2395112281 -144801.803176237;-0.00084 8.78686998685815e-08 -27786.230839122 -145467.493535174;-0.00078 8.66883259425982e-08 -24489.0062178881 -146058.760036488;-0.00072 8.54636006672466e-08 -21179.2525685683 -146575.300177311;-0.00066 8.41951506346079e-08 -17858.6632222869 -147016.849686164;-0.0006 8.2883624807157e-08 -14528.9370539107 -147383.182658159;-0.00054 8.15296941857414e-08 -11191.7776128739 -147674.111670577;-0.00048 8.01340514662849e-08 -7848.89225161008 -147889.487878761;-0.00042 7.86974106853912e-08 -4501.99125203948 -148029.201092262;-0.00036 7.722050685503e-08 -1152.78695055709 -148093.17983122;-0.0003 7.57040955864907e-08 2197.00713803025 -148081.391362928;-0.00024 7.41489527037986e-08 5545.67719716975 -147993.841718586;-0.00018 7.25558738467881e-08 8891.50998538285 -147830.575690209;-0.00012 7.09256740640392e-08 12232.7937127912 -147591.676807714;-6e-05 6.92591873958833e-08 15567.8189169001 -147277.267296183]  x3=[-0.00192 3.79021771114528e-10 0 0;-0.00186 3.77650186609104e-10 0 0;-0.0018 3.76085389290038e-10 0 0;-0.00174 3.74328179736552e-10 0 0;-0.00168 3.72379456969523e-10 0 0;-0.00162 3.70240217991528e-10 0 0;-0.00156 3.67911557276755e-10 0 0;-0.0015 3.65394666211056e-10 0 0;-0.00144 3.62690832482406e-10 0 0;-0.00138 3.59801439422102e-10 0 0;-0.00132 3.56727965297023e-10 0 0;-0.00126 3.53471982553324e-10 0 0;-0.0012 3.50035157011939e-10 0 0;-0.00114 3.46419247016321e-10 -1695.56902120927 -6367.45842345786;-0.00108 3.42626102532837e-10 -1551.11903861574 -6404.17991399322;-0.00102 3.38657664204295e-10 -1405.87547486066 -6437.62490774894;-0.00096 3.34515962357072e-10 -1259.91263923505 -6467.77629364822;-0.0009 3.30203115962363e-10 -1113.3052090227 -6494.61864568491;-0.00084 3.25721331552076e-10 -966.128191293894 -6518.13823081571;-0.00078 3.21072902089928e-10 -818.45688453043 -6538.32301598628;-0.00072 3.16260205798326e-10 -670.366840101496 -6555.16267428755;-0.00066 3.11285704941621e-10 -521.933823610211 -6568.64859023917;-0.0006 3.06151944566369e-10 -373.233776130538 -6578.77386419736;-0.00054 3.00861551199239e-10 -224.34277535443 -6585.53331588487;-0.00048 2.95417231503234e-10 -75.3369966690725 -6588.9234870413;-0.00042 2.89821770892909e-10 73.7073258158483 -6588.94264319245;-0.00036 2.84078032109305e-10 222.713938270927 -6585.59077453768;-0.0003 2.78188953755314e-10 371.606606159906 -6578.86959595494;-0.00024 2.72157548792242e-10 520.309153242673 -6568.78254612337;-0.00018 2.65986902998315e-10 668.745500548433 -6555.33478576406;-0.00012 2.5968017338994e-10 816.839705299117 -6538.53319499969;-6e-05 2.53240586606522e-10 964.515999763107 -6518.38636983456]  x4=[-0.00192 1.28835376332807e-09 0 0;-0.00186 1.29044138525956e-09 0 0;-0.0018 1.29186879353373e-09 0 0;-0.00174 1.29263525786214e-09 0 0;-0.00168 1.29274038610747e-09 0 0;-0.00162 1.29218412448418e-09 0 0;-0.00156 1.29096675758598e-09 0 0;-0.0015 1.28908890824028e-09 0 0;-0.00144 1.28655153718949e-09 0 0;-0.00138 1.28335594259955e-09 0 0;-0.00132 1.27950375939567e-09 0 0;-0.00126 1.27499695842598e-09 0 0;-0.0012 1.26983784545312e-09 0 0;-0.00114 1.26402905997463e-09 -3068.11978237031 348.500730099425;-0.00108 1.25757357387248e-09 -3075.21673451761 279.017978413963;-0.00102 1.25047468989264e-09 -3080.74034896005 209.392475975085;-0.00096 1.24273603995535e-09 -3084.68779971442 139.65984447637;-0.0009 1.23436158329689e-09 -3087.05706719198 69.8557604206038;-0.00084 1.22535560444404e-09 -3087.84693923172 0.0159368670203662;-0.00078 1.21572271102198e-09 -3087.05701172049 -69.8238948401589;-0.00072 1.20546783139699e-09 -3084.68768879981 -139.628003352541;-0.00066 1.19459621215498e-09 -3080.74018265906 -209.360675598378;-0.0006 1.18311341541722e-09 -3075.21651291533 -278.98623505404;-0.00054 1.17102531599472e-09 -3068.11950558013 -348.469059996774;-0.00048 1.1583380983825e-09 -3059.45279161354 -417.773601729447;-0.00042 1.14505825359551e-09 -3049.22080506658 -486.864402767905;-0.00036 1.13119257584774e-09 -3037.42878081262 -555.706114981689;-0.0003 1.11674815907613e-09 -3024.08275186917 -624.263517678779;-0.00024 1.10173239331121e-09 -3009.18954631123 -692.501535625161;-0.00018 1.08615296089619e-09 -2992.75678377798 -760.38525698996;-0.00012 1.07001783255658e-09 -2974.79287157435 -827.879951206979;-6e-05 1.05333526332218e-09 -2955.30700036978 -894.951086743498]  x5=0.00186628717108595  V1=[7.602e-19 2.561e-08 2.561e-08;377 377 377;2.359 1.029 -0.5418]  V2=[1.596e-23 1.649e-13 1.649e-13;377 377 377;-0.06951 1.06 -0.5113]  I1=[1.208e-21 2.221e-10 2.221e-10;377 377 377;-2.873 2.204 0.633]  I2=[1.433e-21 2.255e-10 2.255e-10;377 377 377;1.006 -0.507 -2.078]  nHarmo=1  Measurements=None  Decoupling=off  VsMag0=0  VrMag0=0  VsAngle0=0  VrAngle0=0  IsMag0=0  IrMag0=0  IsAngle0=0  IrAngle0=0
      settings: LibrarySourceBlock=sps_lib/Power Grid Elements/Distributed Parameters Line
  MPP8 3100 KVA 17KV : spsSynchronousMachinepuStandardLib/Synchronous Machine pu Standard  PresetModel=No  MechanicalLoad=Mechanical power Pm  ShowDetailedParameters=on  RotorType=Salient-pole  Units=per unit standard parameters  MeasurementBus=off  NominalParameters=[3100e6 17000 60]  Reactances1=[ 1.81, 0.3, 0.23, 1.76, 0.65, 0.25, 0.15 ]  Reactances2=[ 1.305, 0.296, 0.252, 0.474, 0.243, 0.18 ]  dAxisTimeConstants=Short-circuit  qAxisTimeConstants=Open-circuit  TimeConstants1="[ 4.4849  0.0681  0.1  ]"  TimeConstants2=[ 8.0, 0.03, 1.0, 0.07 ]  TimeConstants3="[  4.49  0.0681  0.0513  ]"  TimeConstants4=[ 8.0, 0.03, 0.3371, 0.0295 ]  TimeConstants5=[ 1.01, 0.053, 0.1 ]  TimeConstants6=[ 1.3201, 0.023, 1.0, 0.07 ]  TimeConstants7=[0.012 0.003 0.003]  TimeConstants8=[ 1.3201, 0.0231, 0.3371, 0.0295 ]  StatorResistance=2.8544e-3  Mechanical=[3.5 0 32]  PolePairs=20  InitialConditions=[0 -81.9543 0.907703 0.907703 0.907703 -8.76021 -128.76 111.24 1.25655]  SetSaturation=off  Saturation=[0.6404,0.7127,0.8441,0.9214,0.9956,1.082,1.19,1.316,1.457;0.7,0.7698,0.8872,0.9466,0.9969,1.046,1.1,1.151,1.201]  LoadFlowParameters=[1,0,0,0,0]  TsPowergui=0  TsBlock=-1  IterativeModel=Trapezoidal non iterative  IterativeDiscreteModel=Trapezoidal non iterative  BusType=PV  Pref=2900e6  Qref=0  Qmin=-inf  Qmax=inf  PLF=0  QLF=0
  MPP9 4100 MVA 17KV : spsSynchronousMachinepuStandardLib/Synchronous Machine pu Standard  PresetModel=No  MechanicalLoad=Mechanical power Pm  ShowDetailedParameters=on  RotorType=Salient-pole  Units=per unit standard parameters  MeasurementBus=off  NominalParameters="[4100e6  17000   60]"  Reactances1=[ 1.81, 0.3, 0.23, 1.76, 0.65, 0.25, 0.15 ]  Reactances2=[ 1.305, 0.296, 0.252, 0.474, 0.243, 0.18 ]  dAxisTimeConstants=Short-circuit  qAxisTimeConstants=Open-circuit  TimeConstants1="[ 4.4849  0.0681  0.1  ]"  TimeConstants2=[ 8.0, 0.03, 1.0, 0.07 ]  TimeConstants3="[  4.49  0.0681  0.0513  ]"  TimeConstants4=[ 8.0, 0.03, 0.3371, 0.0295 ]  TimeConstants5=[ 1.01, 0.053, 0.1 ]  TimeConstants6=[ 1.3201, 0.023, 1.0, 0.07 ]  TimeConstants7=[0.012 0.003 0.003]  TimeConstants8=[ 1.3201, 0.0231, 0.3371, 0.0295 ]  StatorResistance=2.8544e-3  Mechanical=[3.5 0 32]  PolePairs=20  InitialConditions=[0 -81.9543 0.907703 0.907703 0.907703 -8.76021 -128.76 111.24 1.25655]  SetSaturation=off  Saturation=[0.6404,0.7127,0.8441,0.9214,0.9956,1.082,1.19,1.316,1.457;0.7,0.7698,0.8872,0.9466,0.9969,1.046,1.1,1.151,1.201]  LoadFlowParameters=[1,0,0,0,0]  TsPowergui=0  TsBlock=-1  IterativeModel=Trapezoidal non iterative  IterativeDiscreteModel=Trapezoidal non iterative  BusType=PV  Pref=3500e6  Qref=0  Qmin=-inf  Qmax=inf  PLF=0  QLF=0
  Regulators 7 : Subsystem
  Regulators 8 : Subsystem
  Regulators 9 : Subsystem
  ATL-a : PMIOPort  Side=Right
  ATL-b : PMIOPort  Port=2  Side=Right
  ATL-c : PMIOPort  Port=3  Side=Right
  ORE-a : PMIOPort  Port=4  Side=Left
  ORE-b : PMIOPort  Port=5  Side=Left
  ORE-c : PMIOPort  Port=6  Side=Left
  wires:
  Regulators 8/2(Vf) -> MPP8 3100 KVA 17KV/2
  MPP8 3100 KVA 17KV/1 -> Regulators 8/1(m)
  Regulators 8/1(Pm) -> MPP8 3100 KVA 17KV/1
  Regulators 7/1(Pm) -> MPP7 2700 MVA 17KV/1
  Regulators 7/2(Vf) -> MPP7 2700 MVA 17KV/2
  Regulators 9/1(Pm) -> MPP9 4100 MVA 17KV/1
  Regulators 9/2(Vf) -> MPP9 4100 MVA 17KV/2
  MPP9 4100 MVA 17KV/1 -> Regulators 9/1(m)
  MPP7 2700 MVA 17KV/1 -> Regulators 7/1(m)
  connections:
  ATL-c/RConn1 -- ATL-CAD 447 km/RConn3
  1320 MVar/LConn2 -- MPP7-BMW 330 km/RConn2 -- "2700 MVA 17KV :650KV Transformer "/LConn2
  1320 MVar/LConn1 -- MPP7-BMW 330 km/RConn1 -- Load Flow Bus1/LConn1 -- "2700 MVA 17KV :650KV Transformer "/LConn1
  Cs FER/RConn3 -- FER-LTN 78 km/LConn3 -- 990 Mvar/LConn3
  MPP8 3100 KVA 17KV/RConn2 -- "3100 MVA 17KV :650KV Transformer "/RConn2 -- 155 MW/LConn2
  1320 MVar/LConn3 -- MPP7-BMW 330 km/RConn3 -- "2700 MVA 17KV :650KV Transformer "/LConn3
  Cs FER/LConn3 -- BMW- FER 131 km/RConn3
  "3100 MVA 17KV :650KV Transformer "/RConn3 -- 155 MW/LConn3 -- MPP8 3100 KVA 17KV/RConn3
  Cs FER/RConn2 -- FER-LTN 78 km/LConn2 -- 990 Mvar/LConn2
  ATL-CAD 447 km/RConn1 -- ATL-a/RConn1
  "3100 MVA 17KV :650KV Transformer "/RConn1 -- MPP8 3100 KVA 17KV/RConn1 -- Load Flow Bus2/LConn1 -- 155 MW/LConn1
  Cs FER/RConn1 -- FER-LTN 78 km/LConn1 -- 990 Mvar/LConn1
  Cs FER/LConn2 -- BMW- FER 131 km/RConn2
  Cs FER/LConn1 -- BMW- FER 131 km/RConn1
  ATL-b/RConn1 -- ATL-CAD 447 km/RConn2
  "2700 MVA 17KV :650KV Transformer "/RConn1 -- 135 MW/LConn1 -- MPP7 2700 MVA 17KV/RConn1 -- Load Flow Bus/LConn1
  "2700 MVA 17KV :650KV Transformer "/RConn2 -- 135 MW/LConn2 -- MPP7 2700 MVA 17KV/RConn2
  "2700 MVA 17KV :650KV Transformer "/RConn3 -- 135 MW/LConn3 -- MPP7 2700 MVA 17KV/RConn3
  "4100 MVA 17KV :650KV Transformer "/LConn1 -- LTN 3/RConn1 -- Load Flow Bus6/LConn1
  "4100 MVA 17KV :650KV Transformer "/LConn2 -- LTN 3/RConn2
  "4100 MVA 17KV :650KV Transformer "/LConn3 -- LTN 3/RConn3
  MPP9 4100 MVA 17KV/RConn1 -- Load Flow Bus4/LConn1 -- 205 MW/LConn1 -- "4100 MVA 17KV :650KV Transformer "/RConn1
  MPP9 4100 MVA 17KV/RConn2 -- 205 MW/LConn2 -- "4100 MVA 17KV :650KV Transformer "/RConn2
  MPP9 4100 MVA 17KV/RConn3 -- 205 MW/LConn3 -- "4100 MVA 17KV :650KV Transformer "/RConn3
  BMW- FER 131 km/LConn1 -- BMW- ORE 215 km/LConn1 -- 660 MVar/LConn1 -- CAD 3/RConn1 -- Load Flow Bus3/LConn1 -- "3100 MVA 17KV :650KV Transformer "/LConn1 -- Cs BMW- MPP8/LConn1
  "3100 MVA 17KV :650KV Transformer "/LConn2 -- BMW- ORE 215 km/LConn2 -- 660 MVar/LConn2 -- Cs BMW- MPP8/LConn2 -- BMW- FER 131 km/LConn2 -- CAD 3/RConn2
  BMW- FER 131 km/LConn3 -- 660 MVar/LConn3 -- BMW- ORE 215 km/LConn3 -- Cs BMW- MPP8/LConn3 -- CAD 3/RConn3 -- "3100 MVA 17KV :650KV Transformer "/LConn3
  Cs BMWN/RConn1 -- MPP7-BMW 330 km/LConn1
  Cs BMWN/RConn2 -- MPP7-BMW 330 km/LConn2
  Cs BMWN/RConn3 -- MPP7-BMW 330 km/LConn3
  BMW 1/RConn1 -- Cs BMWN/LConn1
  BMW 1/RConn2 -- Cs BMWN/LConn2
  BMW 1/RConn3 -- Cs BMWN/LConn3
  Cs BMW- MPP8/RConn1 -- BMW 1/LConn1
  Cs BMW- MPP8/RConn2 -- BMW 1/LConn2
  Cs BMW- MPP8/RConn3 -- BMW 1/LConn3
  ATL-CAD 447 km/LConn1 -- 1980 MVar/LConn1 -- CAD 3/LConn1
  ATL-CAD 447 km/LConn2 -- 1980 MVar/LConn2 -- CAD 3/LConn2
  ATL-CAD 447 km/LConn3 -- Load Flow Bus8/LConn1 -- CAD 3/LConn3 -- 1980 MVar/LConn3
  Cs ORED/RConn1 -- ORE-a/RConn1
  Cs ORED/RConn2 -- ORE-b/RConn1
  Cs ORED/RConn3 -- ORE-c/RConn1
  BMW- ORE 215 km/RConn1 -- Load Flow Bus7/LConn1 -- Cs ORED/LConn1
  BMW- ORE 215 km/RConn2 -- Cs ORED/LConn2
  BMW- ORE 215 km/RConn3 -- Cs ORED/LConn3
  Cs LTNN/RConn1 -- FER-LTN 78 km/RConn1
  Cs LTNN/RConn2 -- FER-LTN 78 km/RConn2
  Cs LTNN/RConn3 -- FER-LTN 78 km/RConn3
  LTN 3/LConn1 -- Cs LTNN/LConn1
  LTN 3/LConn2 -- Cs LTNN/LConn2
  LTN 3/LConn3 -- Cs LTNN/LConn3

== system 35 Bus Network Electricity Transmission Model/PSS_Equation ==
  In1 : Inport
  1 : Constant
  Sum : Sum  Inputs=|++
  wires:
  In1/1 -> Sum/1
  1/1 -> Sum/2
  Sum/1 -> [PSS_modes]
